simulink model "untitled"  (R2020b)
settings: Solver=VariableStepAuto  StartTime=0.0  StopTime=10.0  MaxStep=0.01  RelTol=1e-3
libraries: simulink_extras x1
settings Model: Creator=kaa040803  LastModifiedBy=kaa040803

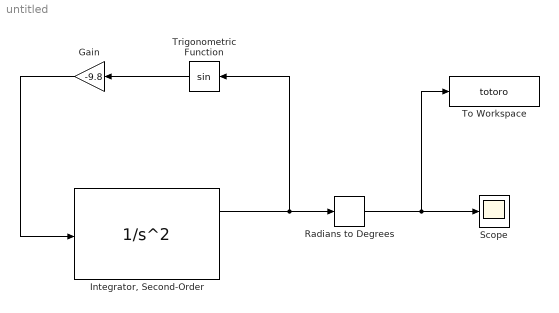
== system untitled ==
  Gain : Gain  Gain=-9.8
  "Integrator, Second-Order" : SecondOrderIntegrator  ICX=55*pi/100
  Radians to Degrees : simulink_extras/Transformations/Radians to Degrees
  Scope : Scope
  To Workspace : ToWorkspace  VariableName=totoro  SampleTime=-1
  Trigonometric Function : Trigonometry
  wires:
  Trigonometric Function/1 -> Gain/1
  "Integrator, Second-Order"/1 -> Radians to Degrees/1, Trigonometric Function/1
  Gain/1 -> "Integrator, Second-Order"/1
  Radians to Degrees/1 -> To Workspace/1, Scope/1
